simulink model "integrated_3PropControl_6bitCmd"  (R2020a)
settings: Solver=FixedStepAuto  StartTime=0.0  StopTime=inf  RelTol=1e-3  EnableMultiTasking=on
undefined symbols (not defined in the file): duplex, Full, Half, RS422, RS485, standard
libraries: xpcseriallib x10, slrtlib x4, simulink x3, speedgoatlib_obsolete x1, speedgoatlib_IO581 x1
settings Model: SimulationMode=external  Creator=MAE-VermillionLab  LastModifiedBy=MAE-VermillionLab
settings SolverCC: ConcurrentTasks=on  AutoInsertRateTranBlk=on
settings DataIOCC: SaveFormat=StructureWithTime
settings OptimizationCC: BlockReduction=off  OptimizeBlockIOStorage=off
settings HardwareCC: ProdBitPerPointer=32  ProdBitPerSizeT=32  ProdBitPerPtrDiffT=32  ProdLargestAtomicFloat=None  ProdWordSize=32  ProdLongLongMode=on  ProdHWDeviceType=Generic->32-bit x86 compatible
settings RTWCC: Description=Simulink Real-Time  SystemTargetFile=slrt.tlc  TemplateMakefile=slrt_default_tmf  CodeExecutionProfiling=on  RTWCompilerOptimization=on
settings SimulinkRealTimeCC: SupportVariableSizeSignals=on  RL32LogTETModifier=off  xPCConcurrentTasks=on

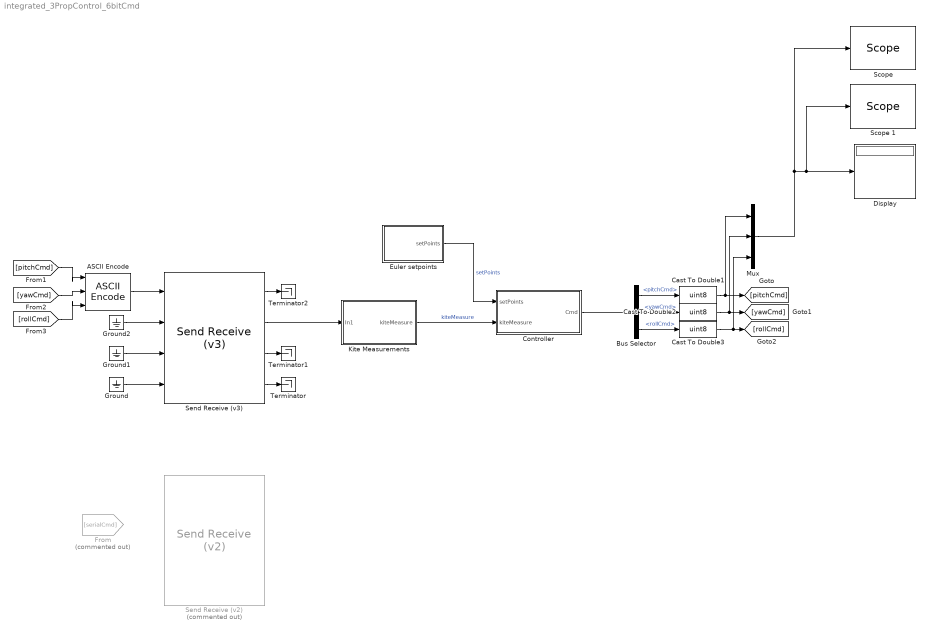
== system integrated_3PropControl_6bitCmd ==
  "ASCII Encode " : xpcseriallib/ASCII Encode   format=%d%d%d  nvars=3  maxlength=256  vartypes={ 'uint8' }
      settings: SourceProductBaseCode=XP
  Bus Selector : BusSelector  OutputSignals=pitchCmd,yawCmd,rollCmd
  Cast To Double1 : DataTypeConversion  OutDataTypeStr=uint8
  Cast To Double2 : DataTypeConversion  OutDataTypeStr=uint8
  Cast To Double3 : DataTypeConversion  OutDataTypeStr=uint8
  Controller : Subsystem  mask{ctrlSurfDefMax=45, pitchKP=1, yawKP=1, rollKP=1}
      mask prompts: ctrlSurfDefMax "Max Ctrlsurf def"; pitchKP "pitch Kp"; yawKP "yaw Kp"; rollKP "roll Kp"
  Display : Display
  "Euler setpoints " : Subsystem  mask{EulerSP=[0 0 0]}
      mask prompts: EulerSP "Euler Setpoints"
  From : From  Commented=on  GotoTag=serialCmd
  Ground : Ground
  Ground1 : Ground
  Ground2 : Ground
  "Kite Measurements " : Subsystem
  Mux : Mux  Inputs=3
  "Scope " : slrtlib/Displays and Logging/Scope   scopeno=1  scopetype=Target  autostart=on  viewmode=Graphical sliding  formatstr='%15.6f'  grid=on  ylimits=[0,100]  nosamples=1000  noprepostsamples=0  interleave=1  triggermode=FreeRun  triggersignal=1  trigsignalfromport=off  triggerlevel=0.0  triggerslope=Either  triggerscope=1  triggersample=0  filename=data.dat  mode=Lazy  writesize=512  autorestart=off  dynamicfilemode=off  maxwritefilesize=512*1024^2
  Scope 1 : slrtlib/Displays and Logging/Scope   scopeno=2  scopetype=Target  autostart=on  viewmode=Numerical  formatstr='%15.6f'  grid=on  ylimits=[-0.5,0.5]  nosamples=1000  noprepostsamples=0  interleave=1  triggermode=FreeRun  triggersignal=1  trigsignalfromport=off  triggerlevel=0.0  triggerslope=Either  triggerscope=1  triggersample=0  filename=data.dat  mode=Lazy  writesize=512  autorestart=off  dynamicfilemode=off  maxwritefilesize=512*1024^2
  Send Receive (v2) : speedgoatlib_obsolete/IO581/Send Receive (v2)  Commented=on  irqnum=5  slot=-1  protocolch12=RS485 (Half-duplex)  protocolch34=RS422 (Full-duplex)  rena1=off  baud1=38400  bauddivisor1=3.125  cstm_baud1=10000000  parity1=None  ndata1=8  nstop1=1  rlevel1=quarter full (64)  hwmode1=none  swmode1=none  xonchar1=17  xoffchar1=19  rs485delay1=0  xmtfifosize1=1024  xmtdatatype1=8 bit uint null terminated  rcvfifosize1=1024  state1=RS485 half-duplex  rena2=off  baud2=38400  bauddivisor2=3.125  cstm_baud2=10000000  parity2=None  ndata2=8  nstop2=1  rlevel2=quarter full (64)  hwmode2=none  swmode2=none  xonchar2=17  xoffchar2=19  rs485delay2=0  xmtfifosize2=1024  xmtdatatype2=8 bit int null terminated  rcvfifosize2=1024  state2=RS485 half-duplex  rena3=off  baud3=2764800  bauddivisor3=3.125  cstm_baud3=10000000  parity3=None  ndata3=8  nstop3=1  rlevel3=1  hwmode3=none  swmode3=none  xonchar3=17  xoffchar3=19  rs485delay3=0  xmtfifosize3=1024  xmtdatatype3=8 bit uint null terminated  rcvfifosize3=1024  state3=RS422  rena4=off  baud4=2764800  bauddivisor4=3.125  cstm_baud4=10000000  parity4=None  ndata4=8  nstop4=1  rlevel4=1  hwmode4=none  swmode4=none  xonchar4=17  xoffchar4=19  rs485delay4=0  xmtfifosize4=1024  xmtdatatype4=8 bit uint null terminated  rcvfifosize4=1024  state4=RS422
      settings: SourceProductName=Simulink Real-Time: Speedgoat Library
  "Send Receive (v3) " : speedgoatlib_IO581/Send Receive (v3)   parModuleId=1  parSlot=-1  parModuleType=IO581  parTransceiver12=RS485 Half-Duplex  parTransceiver34=RS232  parTransceiver1=RS485 Half-Duplex  parAutoTurnaround1=off  parTurnaroundDelay1=0  parStandardBaud1=on  parBaudrate1=38400  parBaudDivisor1=1  parSamplingRate1=16x (standard)  parPrescale1=off  parCalcBaud1=7812500  parParity1=None  parDataBits1=8  parStopBits1=1  parTxTrigLvl1=1  parRxTrigLvl1=1  parHandshake1=none  parRtsHysteresis1=0  parXon1=17  parXoff1=19  parTxSwFifoSize1=1024  parTxSwFifoType1=8 bit uint null terminated  parRxSwFifoSize1=1024  parTransceiver2=RS485 Half-Duplex  parAutoTurnaround2=off  parTurnaroundDelay2=0  parStandardBaud2=on  parBaudrate2=38400  parBaudDivisor2=1  parSamplingRate2=16x (standard)  parPrescale2=off  parCalcBaud2=7812500  parParity2=None  parDataBits2=8  parStopBits2=1  parTxTrigLvl2=1  parRxTrigLvl2=1  parHandshake2=none  parRtsHysteresis2=0  parXon2=17  parXoff2=19  parTxSwFifoSize2=1024  parTxSwFifoType2=8 bit int null terminated  parRxSwFifoSize2=1024  parTransceiver3=RS232  parAutoTurnaround3=off  parTurnaroundDelay3=0  parStandardBaud3=on  parBaudrate3=115200  parBaudDivisor3=1  parSamplingRate3=16x (standard)  parPrescale3=off  parCalcBaud3=7812500  parParity3=None  parDataBits3=8  parStopBits3=1  parTxTrigLvl3=1  parRxTrigLvl3=1  parHandshake3=none  parRtsHysteresis3=0  parXon3=17  parXoff3=19  parTxSwFifoSize3=1024  parTxSwFifoType3=8 bit uint null terminated  parRxSwFifoSize3=1024  parTransceiver4=RS232  parAutoTurnaround4=off  parTurnaroundDelay4=0  parStandardBaud4=on  parBaudrate4=115200  parBaudDivisor4=1  parSamplingRate4=16x (standard)  parPrescale4=off  parCalcBaud4=7812500  parParity4=None  parDataBits4=8  parStopBits4=1  parTxTrigLvl4=1  parRxTrigLvl4=1  parHandshake4=none  parRtsHysteresis4=0  parXon4=17  parXoff4=19  parTxSwFifoSize4=1024  parTxSwFifoType4=8 bit uint null terminated  parRxSwFifoSize4=1024
      settings: SourceProductName=Simulink Real-Time: Speedgoat Library
  Terminator : Terminator
  Terminator1 : Terminator
  Terminator2 : Terminator
  wires:
  "Euler setpoints "/1(setPoints) -> Controller/1(setPoints)  "setPoints"
  "Kite Measurements "/1(kiteMeasure) -> Controller/2(kiteMeasure)  "kiteMeasure"
  "Send Receive (v3) "/1 -> Terminator2/1
  "Send Receive (v3) "/2 -> "Kite Measurements "/1(In1)
  "Send Receive (v3) "/3 -> Terminator1/1
  "Send Receive (v3) "/4 -> Terminator/1
  Ground/1 -> "Send Receive (v3) "/4
  Ground2/1 -> "Send Receive (v3) "/2
  Ground1/1 -> "Send Receive (v3) "/3
  "ASCII Encode "/1 -> "Send Receive (v3) "/1
  Controller/1(Cmd) -> Bus Selector/1
  Bus Selector/1 -> Cast To Double1/1  "<pitchCmd>"
  Bus Selector/2 -> Cast To Double2/1  "<yawCmd>"
  Bus Selector/3 -> Cast To Double3/1  "<rollCmd>"
  Cast To Double1/1 -> Mux/1, [pitchCmd]
  Cast To Double3/1 -> Mux/3, [rollCmd]
  Cast To Double2/1 -> Mux/2, [yawCmd]
  [pitchCmd] -> "ASCII Encode "/1
  [yawCmd] -> "ASCII Encode "/2
  [rollCmd] -> "ASCII Encode "/3
  Mux/1 -> "Scope "/1, Scope 1/1, Display/1

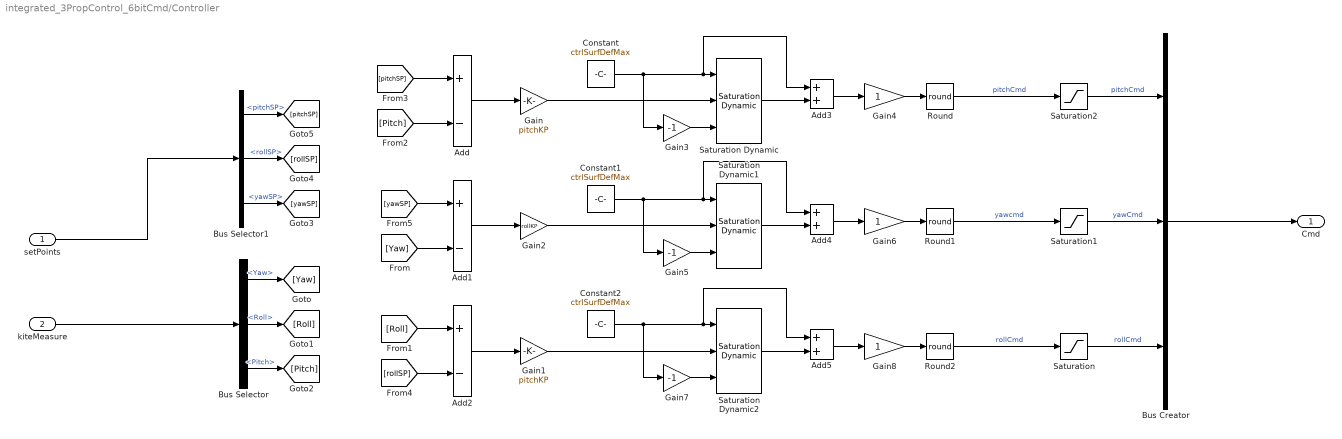
== system integrated_3PropControl_6bitCmd/Controller ==
  setPoints : Inport
  kiteMeasure : Inport  Port=2
  Add : Sum  Inputs=+-
  Add1 : Sum  Inputs=+-
  Add2 : Sum  Inputs=+-
  Add3 : Sum
  Add4 : Sum
  Add5 : Sum
  Bus Creator : BusCreator  Inputs=3
  Bus Selector : BusSelector  OutputSignals=Yaw,Roll,Pitch
  Bus Selector1 : BusSelector  OutputSignals=pitchSP,rollSP,yawSP
  Constant : Constant  Value=ctrlSurfDefMax
  Constant1 : Constant  Value=ctrlSurfDefMax
  Constant2 : Constant  Value=ctrlSurfDefMax
  Gain : Gain  Gain=pitchKP
  Gain1 : Gain  Gain=pitchKP
  Gain2 : Gain  Gain=rollKP
  Gain3 : Gain  Gain=-1
  Gain4 : Gain
  Gain5 : Gain  Gain=-1
  Gain6 : Gain
  Gain7 : Gain  Gain=-1
  Gain8 : Gain
  Round : Rounding  Operator=round
  Round1 : Rounding  Operator=round
  Round2 : Rounding  Operator=round
  Saturation : Saturate  UpperLimit=99  LowerLimit=10
  Saturation Dynamic : simulink/Discontinuities/Saturation Dynamic  OutMin=[]  OutMax=[]  OutDataTypeStr=Inherit: Same as second input  OutDataType=fixdt(1, 16)  OutScaling=2^-10  DoSatur=off
  Saturation Dynamic1 : simulink/Discontinuities/Saturation Dynamic  OutMin=[]  OutMax=[]  OutDataTypeStr=Inherit: Same as second input  OutDataType=fixdt(1, 16)  OutScaling=2^-10  DoSatur=off
  Saturation Dynamic2 : simulink/Discontinuities/Saturation Dynamic  OutMin=[]  OutMax=[]  OutDataTypeStr=Inherit: Same as second input  OutDataType=fixdt(1, 16)  OutScaling=2^-10  DoSatur=off
  Saturation1 : Saturate  UpperLimit=99  LowerLimit=10
  Saturation2 : Saturate  UpperLimit=99  LowerLimit=10
  Cmd : Outport
  wires:
  [Pitch] -> Add/2
  Constant/1 -> Gain3/1, Add3/1, Saturation Dynamic/1
  Bus Selector1/2 -> [rollSP]  "<rollSP>"
  Bus Selector/2 -> [Roll]  "<Roll>"
  Add2/1 -> Gain1/1
  Bus Selector1/1 -> [pitchSP]  "<pitchSP>"
  [Yaw] -> Add1/2
  [rollSP] -> Add2/2
  [yawSP] -> Add1/1
  Add/1 -> Gain/1
  Bus Selector/1 -> [Yaw]  "<Yaw>"
  Gain7/1 -> Saturation Dynamic2/3
  Constant2/1 -> Gain7/1, Add5/1, Saturation Dynamic2/1
  Add5/1 -> Gain8/1
  Gain2/1 -> Saturation Dynamic1/2
  Add1/1 -> Gain2/1
  Add3/1 -> Gain4/1
  Gain5/1 -> Saturation Dynamic1/3
  [Roll] -> Add2/1
  Bus Selector/3 -> [Pitch]  "<Pitch>"
  Saturation Dynamic/1 -> Add3/2
  Bus Selector1/3 -> [yawSP]  "<yawSP>"
  Saturation Dynamic2/1 -> Add5/2
  [pitchSP] -> Add/1
  Gain3/1 -> Saturation Dynamic/3
  Gain4/1 -> Round/1
  Gain8/1 -> Round2/1
  Gain1/1 -> Saturation Dynamic2/2
  Gain6/1 -> Round1/1
  Constant1/1 -> Gain5/1, Add4/1, Saturation Dynamic1/1
  kiteMeasure/1 -> Bus Selector/1
  Saturation Dynamic1/1 -> Add4/2
  Add4/1 -> Gain6/1
  setPoints/1 -> Bus Selector1/1
  Gain/1 -> Saturation Dynamic/2
  Round/1 -> Saturation2/1  "pitchCmd"
  Round1/1 -> Saturation1/1  "yawcmd"
  Round2/1 -> Saturation/1  "rollCmd"
  Saturation2/1 -> Bus Creator/1  "pitchCmd"
  Saturation1/1 -> Bus Creator/2  "yawCmd"
  Saturation/1 -> Bus Creator/3  "rollCmd"
  Bus Creator/1 -> Cmd/1

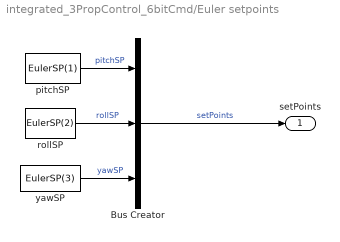
== system integrated_3PropControl_6bitCmd/Euler setpoints  ==
  Bus Creator : BusCreator  Inputs=3
  pitchSP : Constant  Value=EulerSP(1)
  rollSP : Constant  Value=EulerSP(2)
  yawSP : Constant  Value=EulerSP(3)
  setPoints : Outport
  wires:
  rollSP/1 -> Bus Creator/2  "rollSP"
  yawSP/1 -> Bus Creator/3  "yawSP"
  pitchSP/1 -> Bus Creator/1  "pitchSP"
  Bus Creator/1 -> setPoints/1  "setPoints"

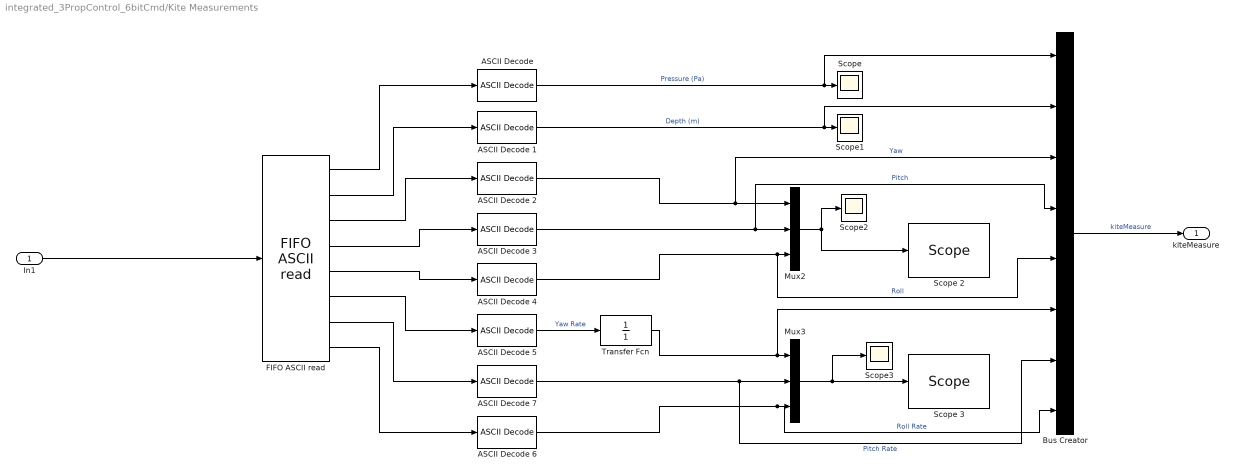
== system integrated_3PropControl_6bitCmd/Kite Measurements  ==
  In1 : Inport
  "ASCII Decode " : xpcseriallib/ASCII Decode   format=p %f\r\n  nvars=1  vartypes={}
      settings: SourceProductBaseCode=XP
  ASCII Decode 1 : xpcseriallib/ASCII Decode   format=d %f\r\n  nvars=1  vartypes={}
      settings: SourceProductBaseCode=XP
  ASCII Decode 2 : xpcseriallib/ASCII Decode   format=x %f\r\n  nvars=1  vartypes={}
      settings: SourceProductBaseCode=XP
  ASCII Decode 3 : xpcseriallib/ASCII Decode   format=y %f\r\n  nvars=1  vartypes={}
      settings: SourceProductBaseCode=XP
  ASCII Decode 4 : xpcseriallib/ASCII Decode   format=z %f\r\n  nvars=1  vartypes={}
      settings: SourceProductBaseCode=XP
  ASCII Decode 5 : xpcseriallib/ASCII Decode   format=wx %f\r\n  nvars=1  vartypes={}
      settings: SourceProductBaseCode=XP
  ASCII Decode 6 : xpcseriallib/ASCII Decode   format=wz %f\r\n  nvars=1  vartypes={}
      settings: SourceProductBaseCode=XP
  ASCII Decode 7 : xpcseriallib/ASCII Decode   format=wy %f\r\n  nvars=1  vartypes={}
      settings: SourceProductBaseCode=XP
  Bus Creator : BusCreator  Inputs=8
  "FIFO ASCII read " : xpcseriallib/FIFO ASCII read   header={'p','d','x','y','z','wx','wy','wz'}  term=[13 10]  hold=Zero output if no new data  enable=off  maxsize=1024  outputtype=8 bit uint null terminated  sampletime=0.01
      settings: SourceProductBaseCode=XP
  Mux2 : Mux  Inputs=3
  Mux3 : Mux  Inputs=3
  Scope{,1..3} (4 alike) : Scope
  Scope 2 : slrtlib/Displays and Logging/Scope   scopeno=3  scopetype=Target  autostart=on  viewmode=Graphical sliding  formatstr='%15.6f'  grid=on  ylimits=[-90,90]  nosamples=1000  noprepostsamples=0  interleave=1  triggermode=FreeRun  triggersignal=1  trigsignalfromport=off  triggerlevel=0.0  triggerslope=Either  triggerscope=1  triggersample=0  filename=data.dat  mode=Lazy  writesize=512  autorestart=off  dynamicfilemode=off  maxwritefilesize=512*1024^2
  Scope 3 : slrtlib/Displays and Logging/Scope   scopeno=4  scopetype=Target  autostart=on  viewmode=Graphical rolling  formatstr='%15.6f'  grid=on  ylimits=[-50,50]  nosamples=1000  noprepostsamples=0  interleave=1  triggermode=FreeRun  triggersignal=1  trigsignalfromport=off  triggerlevel=0.0  triggerslope=Either  triggerscope=1  triggersample=0  filename=data.dat  mode=Lazy  writesize=512  autorestart=off  dynamicfilemode=off  maxwritefilesize=512*1024^2
  Transfer Fcn : TransferFcn  Denominator=[1]
  kiteMeasure : Outport
  wires:
  "FIFO ASCII read "/4 -> ASCII Decode 3/1
  ASCII Decode 2/1 -> Mux2/1, Bus Creator/3  "Yaw"
  ASCII Decode 3/1 -> Mux2/2, Bus Creator/4  "Pitch"
  ASCII Decode 6/1 -> Bus Creator/8, Mux3/3  "Roll Rate"
  ASCII Decode 1/1 -> Bus Creator/2, Scope1/1  "Depth (m)"
  "ASCII Decode "/1 -> Bus Creator/1, Scope/1  "Pressure (Pa)"
  ASCII Decode 7/1 -> Mux3/2, Bus Creator/7  "Pitch Rate"
  "FIFO ASCII read "/1 -> "ASCII Decode "/1
  ASCII Decode 5/1 -> Transfer Fcn/1  "Yaw Rate"
  Mux3/1 -> Scope 3/1, Scope3/1
  "FIFO ASCII read "/5 -> ASCII Decode 4/1
  "FIFO ASCII read "/3 -> ASCII Decode 2/1
  ASCII Decode 4/1 -> Bus Creator/5, Mux2/3  "Roll"
  "FIFO ASCII read "/7 -> ASCII Decode 7/1
  Mux2/1 -> Scope 2/1, Scope2/1
  "FIFO ASCII read "/8 -> ASCII Decode 6/1
  "FIFO ASCII read "/6 -> ASCII Decode 5/1
  "FIFO ASCII read "/2 -> ASCII Decode 1/1
  Bus Creator/1 -> kiteMeasure/1  "kiteMeasure"
  In1/1 -> "FIFO ASCII read "/1
  Transfer Fcn/1 -> Bus Creator/6, Mux3/1
